simulink model "sampleModel1438_sub_sub"  (R2023a)
settings: Solver=VariableStepAuto  StartTime=0.0  StopTime=10.0  RelTol=1e-3
libraries: hdlsllib x4, simulink x1
settings Model: Creator=user1  LastModifiedBy=user1
settings OptimizationCC: BlockReduction=off  ConditionallyExecuteInputs=off

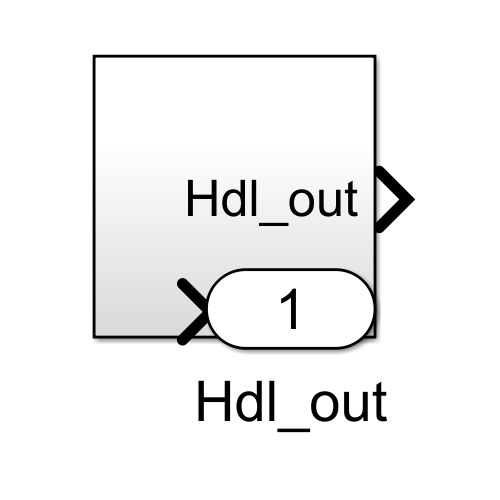
[thumbnail: Simulink's stored preview of the top-level diagram]
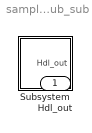
== system sampleModel1438_sub_sub ==
  Subsystem : Subsystem
  Hdl_out : Outport  OutDataTypeStr=uint8

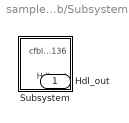
== system sampleModel1438_sub_sub/Subsystem ==
  Subsystem : Subsystem
  Hdl_out : Outport  OutDataTypeStr=uint8

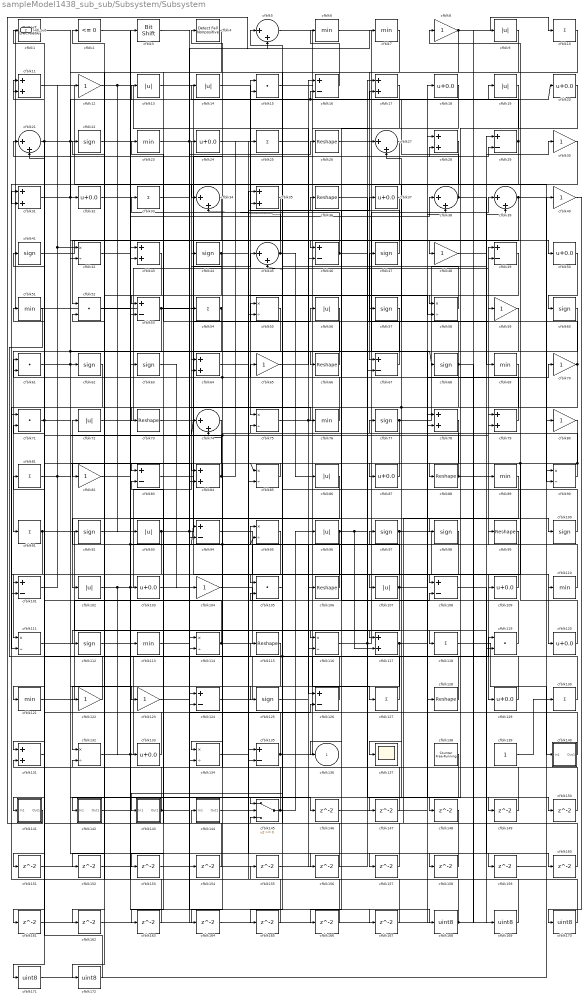
== system sampleModel1438_sub_sub/Subsystem/Subsystem ==
  cfblk1 : simulink/Logic and Bit Operations/Detect Decrease  vinit=0.0  OutDataTypeStr=uint8
      settings: LibrarySourceBlock=|
      | hdlsllib/Logic and Bit
      | Operations/Detect
      | Decrease
  cfblk{10,25,33,54,81,91,118,127,130} (9 alike) : Sum  Inputs=+  OutDataTypeStr=uint8
  cfblk{22,41,44,47,57,60,62..63,68,77,92,97..98,100,112,125} (16 alike) : Signum
  cfblk{16,29,46,49,53,67,83,94,101,108,124,126,135} (13 alike) : Sum  Inputs=+-  OutDataTypeStr=uint8
  cfblk{9,13..14,19,56,72,86,93,96,102,107} (11 alike) : Abs  OutDataTypeStr=uint8  SaturateOnIntegerOverflow=off
  cfblk{18,20,24,32,37,50,87,103,109,120,129,133} (12 alike) : Bias  Bias=0.0  SaturateOnIntegerOverflow=off
  cfblk{8,12,30,40,48,59,65,70,80,82,104,122..123} (13 alike) : Gain  OutDataTypeStr=uint8
  cfblk{15,52,61,71,105,119} (6 alike) : DotProduct  OutDataTypeStr=uint8
  cfblk{26,36,66,73,88,99,106,115,128} (9 alike) : Reshape
  cfblk{11,17,28,31,35,43,64,78..79,84,117,131} (12 alike) : Sum  OutDataTypeStr=uint8
  cfblk{6..7,23,51,69,76,89,110,113,121} (10 alike) : MinMax  OutDataTypeStr=uint8
  cfblk{42,55,58,75,85,90,95,111,114,116,132,134} (12 alike) : Product  Inputs=*/  OutDataTypeStr=uint8  RndMeth=Zero  SaturateOnIntegerOverflow=on
  cfblk137 : Scope
  cfblk138 : hdlsllib/Sources/Counter Free-Running  NumBits=16  tsamp=-1
  cfblk139 : Constant  OutDataTypeStr=uint8  SampleTime=-1
  cfblk140 : Subsystem
      settings: LibrarySourceBlock=|
      | hdlsllib/Ports &
      | Subsystems/Subsystem
  cfblk141 : Subsystem
      settings: LibrarySourceBlock=|
      | hdlsllib/Ports &
      | Subsystems/Subsystem
  cfblk142 : Subsystem
      settings: LibrarySourceBlock=|
      | hdlsllib/Ports &
      | Subsystems/Subsystem
  cfblk143 : Subsystem
      settings: LibrarySourceBlock=|
      | hdlsllib/Ports &
      | Subsystems/Subsystem
  cfblk144 : Subsystem
      settings: LibrarySourceBlock=|
      | hdlsllib/Ports &
      | Subsystems/Subsystem
  cfblk145 : Switch  OutDataTypeStr=uint8  SaturateOnIntegerOverflow=off  InputSameDT=off
  cfblk{146..167} (22 alike) : Delay  SampleTime=1
  cfblk{168..172} (5 alike) : DataTypeConversion  OutDataTypeStr=uint8  SaturateOnIntegerOverflow=off  RndMeth=Floor
  cfblk2 : hdlsllib/Logic and Bit Operations/Compare To Zero  relop=<=  OutDataTypeStr=uint8
  cfblk{5,21,27,34,38..39,45,74} (8 alike) : Sum  Inputs=|++  OutDataTypeStr=uint8
  cfblk3 : hdlsllib/Logic and Bit Operations/Bit Shift  mode=Shift Left Logical  N=0
  cfblk4 : hdlsllib/Logic and Bit Operations/Detect Fall Nonpositive  vinit=0  OutDataTypeStr=uint8
  cfblk136 : Outport  OutDataTypeStr=uint8  VectorParamsAs1DForOutWhenUnconnected=off
  Hdl_out : Outport  Port=2  OutDataTypeStr=uint8
  wires:
  cfblk172/1 -> cfblk71/2
  cfblk138/1 -> cfblk172/1
  cfblk171/1 -> cfblk40/1
  cfblk170/1 -> cfblk71/1
  cfblk40/1 -> cfblk170/1
  cfblk169/1 -> cfblk2/1
  cfblk168/1 -> cfblk155/1, cfblk9/1
  cfblk167/1 -> cfblk145/2
  cfblk103/1 -> cfblk167/1
  cfblk166/1 -> cfblk135/1
  cfblk17/1 -> cfblk166/1
  cfblk165/1 -> cfblk43/1
  cfblk57/1 -> cfblk165/1
  cfblk164/1 -> cfblk38/2
  cfblk163/1 -> cfblk31/1
  cfblk162/1 -> cfblk114/1
  cfblk99/1 -> cfblk162/1
  cfblk161/1 -> cfblk39/2
  cfblk160/1 -> cfblk52/2
  cfblk108/1 -> cfblk160/1
  cfblk159/1 -> cfblk90/1
  cfblk92/1 -> cfblk159/1
  cfblk158/1 -> cfblk83/2
  cfblk157/1 -> cfblk124/1
  cfblk24/1 -> cfblk157/1
  cfblk156/1 -> cfblk105/2
  cfblk155/1 -> cfblk67/2
  cfblk154/1 -> cfblk131/2
  cfblk33/1 -> cfblk154/1
  cfblk153/1 -> cfblk116/2
  cfblk34/1 -> cfblk153/1
  cfblk152/1 -> cfblk85/2
  cfblk95/1 -> cfblk152/1
  cfblk151/1 -> cfblk94/2
  cfblk150/1 -> cfblk1/1
  cfblk149/1 -> cfblk35/1
  cfblk36/1 -> cfblk149/1
  cfblk148/1 -> cfblk145/3
  cfblk19/1 -> cfblk148/1
  cfblk147/1 -> cfblk132/2
  cfblk28/1 -> cfblk147/1
  cfblk146/1 -> cfblk78/2
  cfblk123/1 -> cfblk114/2
  cfblk25/1 -> cfblk19/1
  cfblk113/1 -> cfblk79/1
  cfblk67/1 -> cfblk35/2
  cfblk15/1 -> cfblk27/1
  cfblk70/1 -> cfblk47/1, cfblk88/1
  cfblk68/1 -> cfblk107/1, cfblk163/1, cfblk89/1, cfblk27/2
  cfblk84/1 -> cfblk61/2, cfblk25/1
  cfblk87/1 -> cfblk84/1
  cfblk115/1 -> cfblk125/1
  cfblk52/1 -> cfblk43/2
  cfblk98/1 -> cfblk134/1
  cfblk39/1 -> cfblk80/1, cfblk136/1
  cfblk8/1 -> cfblk10/1, cfblk42/2
  cfblk23/1 -> cfblk98/1, cfblk7/1
  cfblk1/1 -> cfblk123/1
  cfblk16/1 -> cfblk6/1
  cfblk142/1(Out1) -> cfblk38/1, cfblk95/2
  cfblk45/1 -> cfblk34/2, cfblk86/1
  cfblk143/1(Out1) -> cfblk81/1, cfblk126/2
  cfblk131/1 -> cfblk11/1
  cfblk49/1 -> cfblk53/2
  cfblk130/1 -> cfblk45/2, cfblk74/2
  cfblk129/1 -> cfblk64/2
  cfblk37/1 -> cfblk73/1
  cfblk31/1 -> cfblk68/1, cfblk84/2, cfblk13/1
  cfblk118/1 -> cfblk140/1(In1)
  cfblk88/1 -> cfblk21/1, cfblk169/1
  cfblk134/1 -> cfblk37/1
  cfblk74/1 -> cfblk112/1
  cfblk62/1 -> cfblk121/1
  cfblk53/1 -> cfblk26/1, cfblk151/1
  cfblk140/1(Out1) -> cfblk64/1, cfblk94/1
  cfblk65/1 -> cfblk16/1
  cfblk111/1 -> cfblk3/1
  cfblk80/1 -> cfblk109/1, cfblk171/1
  cfblk64/1 -> cfblk117/1
  cfblk71/1 -> cfblk131/1, cfblk79/2
  cfblk12/1 -> cfblk106/1, cfblk93/1
  cfblk43/1 -> cfblk142/1(In1)
  cfblk81/1 -> cfblk12/1, cfblk156/1
  cfblk94/1 -> cfblk110/1
  cfblk3/1 -> cfblk76/1
  cfblk27/1 -> cfblk46/1
  cfblk133/1 -> cfblk41/1
  cfblk119/1 -> cfblk36/1
  cfblk2/1 -> cfblk168/1
  cfblk7/1 -> cfblk53/1
  cfblk76/1 -> cfblk44/1, cfblk21/2
  cfblk75/1 -> cfblk118/1, cfblk119/2
  cfblk104/1 -> cfblk108/2
  cfblk107/1 -> cfblk70/1, cfblk75/2, cfblk122/1
  cfblk11/1 -> cfblk90/2
  cfblk44/1 -> cfblk124/2, cfblk57/1
  cfblk122/1 -> cfblk51/1
  cfblk141/1(Out1) -> cfblk5/2
  cfblk126/1 -> cfblk54/1, cfblk74/1
  cfblk22/1 -> cfblk103/1
  cfblk4/1 -> cfblk82/1
  cfblk30/1 -> cfblk34/1
  cfblk139/1 -> cfblk130/1
  cfblk128/1 -> cfblk61/1
  cfblk102/1 -> cfblk24/1, cfblk158/1, cfblk133/1
  cfblk38/1 -> cfblk69/1, cfblk17/2
  cfblk79/1 -> cfblk65/1
  cfblk83/1 -> cfblk29/2
  cfblk93/1 -> cfblk45/1, cfblk15/2, cfblk101/1
  cfblk127/1 -> cfblk95/1
  cfblk59/1 -> cfblk135/2
  cfblk125/1 -> cfblk99/1
  cfblk29/1 -> cfblk4/1, cfblk31/2
  cfblk21/1 -> cfblk126/1, cfblk46/2, cfblk161/1
  cfblk135/1 -> cfblk17/1, cfblk22/1
  cfblk61/1 -> cfblk62/1, cfblk146/1
  cfblk60/1 -> cfblk137/1
  cfblk145/1 -> cfblk14/1, cfblk96/1
  cfblk32/1 -> cfblk100/1
  cfblk26/1 -> cfblk128/1
  cfblk48/1 -> cfblk30/1
  cfblk66/1 -> cfblk23/1
  cfblk112/1 -> cfblk63/1
  cfblk18/1 -> cfblk66/1
  cfblk9/1 -> cfblk105/1
  cfblk54/1 -> cfblk92/1, Hdl_out/1
  cfblk97/1 -> cfblk120/1, cfblk134/2
  cfblk82/1 -> cfblk20/1, cfblk16/2
  cfblk20/1 -> cfblk58/1
  cfblk58/1 -> cfblk5/1
  cfblk13/1 -> cfblk129/1
  cfblk124/1 -> cfblk18/1
  cfblk144/1(Out1) -> cfblk55/2
  cfblk132/1 -> cfblk78/1, cfblk119/1
  cfblk90/1 -> cfblk85/1, cfblk77/1
  cfblk100/1 -> cfblk55/1
  cfblk46/1 -> cfblk33/1, cfblk58/2
  cfblk121/1 -> cfblk28/1
  cfblk109/1 -> cfblk108/1
  cfblk55/1 -> cfblk141/1(In1)
  cfblk42/1 -> cfblk113/1
  cfblk14/1 -> cfblk75/1
  cfblk78/1 -> cfblk87/1
  cfblk51/1 -> cfblk115/1
  cfblk96/1 -> cfblk59/1, cfblk117/2, cfblk111/1
  cfblk56/1 -> cfblk91/1
  cfblk86/1 -> cfblk102/1
  cfblk106/1 -> cfblk72/1
  cfblk73/1 -> cfblk56/1
  cfblk41/1 -> cfblk50/1
  cfblk117/1 -> cfblk132/1, cfblk150/1
  cfblk110/1 -> cfblk49/2
  cfblk10/1 -> cfblk67/1
  cfblk89/1 -> cfblk144/1(In1)
  cfblk77/1 -> cfblk29/1, cfblk164/1
  cfblk91/1 -> cfblk116/1, cfblk101/2
  cfblk6/1 -> cfblk48/1
  cfblk85/1 -> cfblk83/1
  cfblk50/1 -> cfblk60/1
  cfblk105/1 -> cfblk143/1(In1)
  cfblk114/1 -> cfblk97/1, cfblk11/2
  cfblk116/1 -> cfblk39/1, cfblk28/2
  cfblk72/1 -> cfblk49/1
  cfblk120/1 -> cfblk8/1
  cfblk35/1 -> cfblk52/1
  cfblk101/1 -> cfblk32/1, cfblk42/1
  cfblk47/1 -> cfblk15/1
  cfblk69/1 -> cfblk145/1, cfblk111/2
  cfblk63/1 -> cfblk104/1
  cfblk5/1 -> cfblk127/1

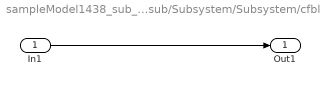
== system sampleModel1438_sub_sub/Subsystem/Subsystem/cfblk140 ==
  In1 : Inport
  Out1 : Outport
  wires:
  In1/1 -> Out1/1

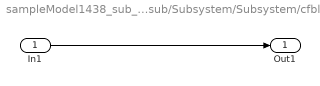
== system sampleModel1438_sub_sub/Subsystem/Subsystem/cfblk141 ==
  In1 : Inport
  Out1 : Outport
  wires:
  In1/1 -> Out1/1

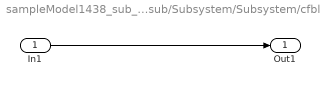
== system sampleModel1438_sub_sub/Subsystem/Subsystem/cfblk142 ==
  In1 : Inport
  Out1 : Outport
  wires:
  In1/1 -> Out1/1

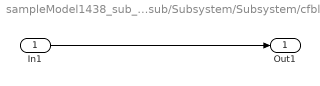
== system sampleModel1438_sub_sub/Subsystem/Subsystem/cfblk143 ==
  In1 : Inport
  Out1 : Outport
  wires:
  In1/1 -> Out1/1

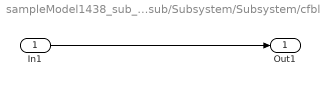
== system sampleModel1438_sub_sub/Subsystem/Subsystem/cfblk144 ==
  In1 : Inport
  Out1 : Outport
  wires:
  In1/1 -> Out1/1
